simulink model "AM_FM"  (R2023a)
settings: Solver=VariableStepAuto  StartTime=0.0  StopTime=0.5  RelTol=1e-3
libraries: commanabbnd3 x4, dspfdesign x1, commsynccomp2 x1
settings Model: SimulationMode=accelerator  Creator=moleiva  LastModifiedBy=luisc
settings ModelReferenceCC: EnableRefExpFcnMdlSchedulingChecks=on

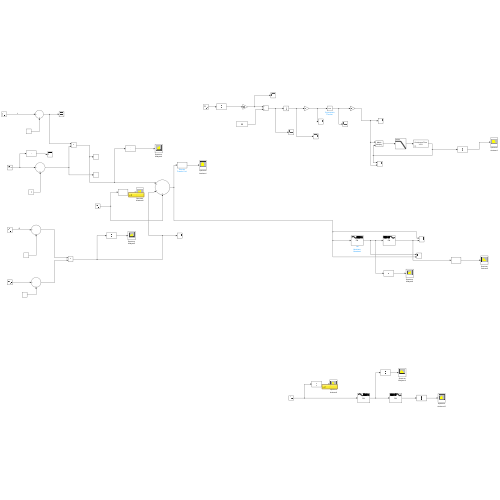
[thumbnail: Simulink's stored preview of the top-level diagram]
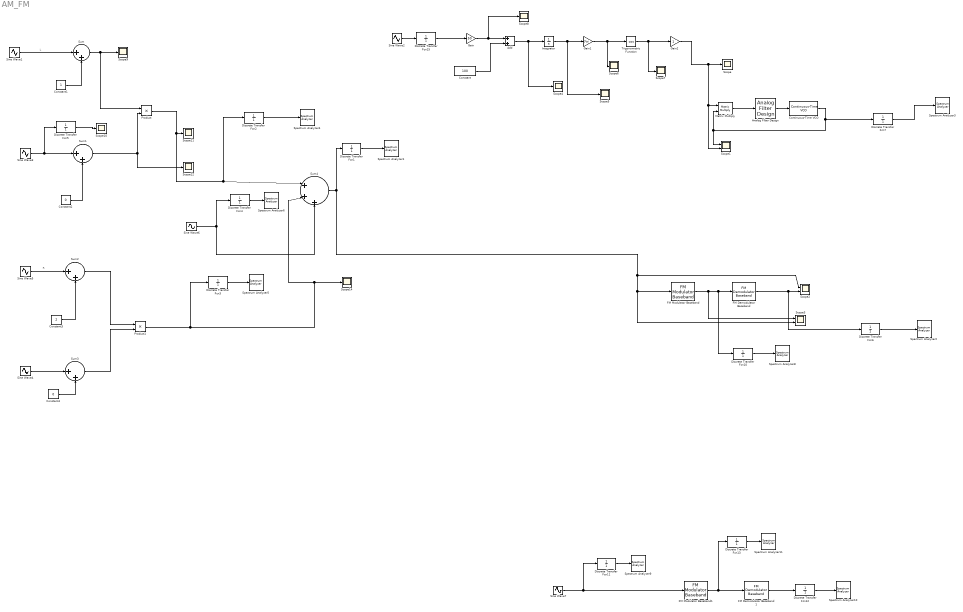
== system AM_FM ==
  note: R
  note: L
  Add : Sum
  Analog Filter Design : dspfdesign/Analog Filter Design  method=Butterworth  filttype=Lowpass  N=8  Wlo=20e+6  Whi=80  Rp=2  Rs=40
  Constant : Constant  Value=100  VectorParams1D=off
  Constant1 : Constant
  Constant2 : Constant  Value=0
  Constant3 : Constant  Value=2
  Constant4 : Constant  Value=0
  Continuous-Time VCO : commsynccomp2/Continuous-Time VCO  Ac=1  Fc=10  Kc=1  Ph=0
  Discrete Transfer Fcn1 : DiscreteTransferFcn  Denominator=[1]  SampleTime=1/24e+6
  Discrete Transfer Fcn{2,5..6,10,12} (5 alike) : DiscreteTransferFcn  Denominator=[1]  SampleTime=1/16e+6
  Discrete Transfer Fcn11 : DiscreteTransferFcn  Denominator=[1]  SampleTime=1/12e+6
  Discrete Transfer Fcn13 : DiscreteTransferFcn  Denominator=[1]  SampleTime=1/12e+6
  Discrete Transfer Fcn15 : DiscreteTransferFcn  Denominator=[1]  SampleTime=1/2*pi*100
  Discrete Transfer Fcn3 : DiscreteTransferFcn  Denominator=[1]  SampleTime=1/24e+6
  Discrete Transfer Fcn4 : DiscreteTransferFcn  Denominator=[1]  SampleTime=1/12e+6
  Discrete Transfer Fcn7 : DiscreteTransferFcn  Denominator=[1]  SampleTime=1/200
  "FM Demodulator Baseband " : commanabbnd3/FM Demodulator Baseband   FrequencyDeviation=50  SimulateUsing=Code generation
  FM Demodulator Baseband 1 : commanabbnd3/FM Demodulator Baseband   FrequencyDeviation=50  SimulateUsing=Code generation
  FM Modulator Baseband : commanabbnd3/FM Modulator Baseband  FrequencyDeviation=50  SimulateUsing=Code generation
  FM Modulator Baseband1 : commanabbnd3/FM Modulator Baseband  FrequencyDeviation=50  SimulateUsing=Code generation
  Gain : Gain  Gain=50
  Gain1 : Gain  Gain=2*pi
  Gain2 : Gain
  Integrator : Integrator
  Matrix Multiply : Product  Multiplication=Matrix(*)
  Product : Product
  Product1 : Product
  Scope{,4..12,14} (11 alike) : Scope
  Scope1 : Scope  NumInputPorts=2
  Scope2 : Scope  NumInputPorts=2
  Scope3 : Scope  NumInputPorts=2
  Sine Wave1 : Sin  Frequency=2*pi*5000  Phase=pi/2  SampleTime=0  VectorParams1D=off
  Sine Wave2 : Sin  Frequency=2*pi*50  Phase=pi/2  SampleTime=0  VectorParams1D=off
  Sine Wave3 : Sin  Frequency=2*pi*8e+6  Phase=pi/2  SampleTime=0  VectorParams1D=off
  Sine Wave4 : Sin  Frequency=2*pi*12e+6  Phase=pi/2  SampleTime=0  VectorParams1D=off
  Sine Wave5 : Sin  Frequency=2*pi*4000  Phase=pi/2  SampleTime=0  VectorParams1D=off
  Sine Wave6 : Sin  Amplitude=2  Frequency=2*pi*6e+6  Phase=pi/2  SampleTime=0  VectorParams1D=off
  Sine Wave7 : Sin  Amplitude=2  Frequency=2*pi*6e+6  Phase=pi/2  SampleTime=0  VectorParams1D=off
  Spectrum Analyzer1 : SpectrumAnalyzer  WindowPosition=[1.000000,41.000000,1536.000000,801.000000,]  ScopeFrameLocation=window  AxesScaling=Manual  AveragingMethod=Exponential  SpectrumUnits=Watts  YLimits=[-0.51276374,4.61487369]  ShowLegend=on  ChannelNames="[\"\"]"  SelectedToolstripTab=spectrumAnalyzerToolstrip.spectrumTab  DefaultConfigurationName=spbscopes.SpectrumAnalyzerBlockCfg
      settings: OpenAtSimulationStart=off
  Spectrum Analyzer10 : SpectrumAnalyzer  WindowPosition=[770.000000,42.000000,766.000000,793.000000,]  Visible=on  ScopeFrameLocation=window  AxesScaling=Manual  AveragingMethod=Exponential  YLimits=[-73.15760482,41.44536822]  ChannelNames="[\"\"]"  DefaultConfigurationName=spbscopes.SpectrumAnalyzerBlockCfg
      settings: OpenAtSimulationStart=off
  Spectrum Analyzer11 : SpectrumAnalyzer  WindowPosition=[2.000000,42.000000,766.000000,793.000000,]  Visible=on  ScopeFrameLocation=window  AxesScaling=Manual  AveragingMethod=Exponential  YLimits=[-74.13776805,40.75747711]  ChannelNames="[\"\"]"  DefaultConfigurationName=spbscopes.SpectrumAnalyzerBlockCfg
      settings: OpenAtSimulationStart=off
  Spectrum Analyzer2 : SpectrumAnalyzer  WindowPosition=[1.000000,41.000000,1536.000000,801.000000,]  Visible=on  ScopeFrameLocation=window  AxesScaling=Manual  AveragingMethod=Exponential  YLimits=[-221.40437999,59.98570956]  ChannelNames="[\"\"]"  DefaultConfigurationName=spbscopes.SpectrumAnalyzerBlockCfg
      settings: OpenAtSimulationStart=off
  Spectrum Analyzer3 : SpectrumAnalyzer  WindowPosition=[1.000000,41.000000,1536.000000,801.000000,]  ScopeFrameLocation=window  AxesScaling=Manual  AveragingMethod=Exponential  SpectrumUnits=Watts  YLimits=[-123.17973841,46.92856517]  ChannelNames="[\"\"]"  SelectedToolstripTab=spectrumAnalyzerToolstrip.spectrumTab  DefaultConfigurationName=spbscopes.SpectrumAnalyzerBlockCfg
      settings: OpenAtSimulationStart=off
  Spectrum Analyzer4 : SpectrumAnalyzer  WindowPosition=[1.000000,1.000000,1536.000000,841.000000,]  ScopeFrameLocation=window  AxesScaling=Manual  AveragingMethod=Exponential  YLimits=[-149.30305087,57.1601735]  ChannelNames="[\"\"]"  DefaultConfigurationName=spbscopes.SpectrumAnalyzerBlockCfg
      settings: OpenAtSimulationStart=off
  Spectrum Analyzer5 : SpectrumAnalyzer  WindowPosition=[368.000000,182.000000,800.000000,500.000000,]  ScopeFrameLocation=window  AxesScaling=Manual  AveragingMethod=Exponential  ChannelNames="[\"\"]"  DefaultConfigurationName=spbscopes.SpectrumAnalyzerBlockCfg
      settings: OpenAtSimulationStart=off
  Spectrum Analyzer6 : SpectrumAnalyzer  WindowPosition=[368.000000,182.000000,800.000000,500.000000,]  ScopeFrameLocation=window  AxesScaling=Manual  AveragingMethod=Exponential  ChannelNames="[\"\"]"  DefaultConfigurationName=spbscopes.SpectrumAnalyzerBlockCfg
      settings: OpenAtSimulationStart=off
  Spectrum Analyzer8 : SpectrumAnalyzer  WindowPosition=[2.000000,42.000000,1534.000000,793.000000,]  ScopeFrameLocation=window  AxesScaling=Manual  AveragingMethod=Exponential  YLimits=[-117.39798875,29.52252221]  ChannelNames="[\"\"]"  DefaultConfigurationName=spbscopes.SpectrumAnalyzerBlockCfg
      settings: OpenAtSimulationStart=off
  Spectrum Analyzer9 : SpectrumAnalyzer  WindowPosition=[90.000000,154.000000,800.000000,500.000000,]  ScopeFrameLocation=window  AxesScaling=Manual  AveragingMethod=Exponential  ChannelNames="[\"\"]"  DefaultConfigurationName=spbscopes.SpectrumAnalyzerBlockCfg
      settings: OpenAtSimulationStart=off
  Sum{,1..3} (4 alike) : Sum  Inputs=|++
  Sum4 : Sum  Inputs=|+++
  Trigonometric Function : Trigonometry  Operator=cos
  wires:
  Gain/1 -> Scope8/1, Add/1
  Add/1 -> Scope4/1, Integrator/1
  Integrator/1 -> Scope5/1, Gain1/1
  Gain1/1 -> Scope6/1, Trigonometric Function/1
  Trigonometric Function/1 -> Scope7/1, Gain2/1
  Constant/1 -> Add/2
  Gain2/1 -> Scope1/2, Matrix Multiply/1, Scope/1
  Matrix Multiply/1 -> Analog Filter Design/1
  Analog Filter Design/1 -> Continuous-Time VCO/1
  Sum4/1 -> Scope3/2, FM Modulator Baseband/1, Scope2/1, Discrete Transfer Fcn1/1
  FM Modulator Baseband/1 -> Scope3/1, Discrete Transfer Fcn10/1, "FM Demodulator Baseband "/1
  "FM Demodulator Baseband "/1 -> Discrete Transfer Fcn6/1, Scope2/2
  Sum3/1 -> Product1/2
  Discrete Transfer Fcn2/1 -> Spectrum Analyzer4/1
  Discrete Transfer Fcn5/1 -> Scope10/1
  Discrete Transfer Fcn1/1 -> Spectrum Analyzer1/1
  Sum1/1 -> Product/2, Scope12/1
  Sum/1 -> Product/1, Scope9/1
  Discrete Transfer Fcn3/1 -> Spectrum Analyzer5/1
  Constant3/1 -> Sum2/2
  Constant1/1 -> Sum/2
  Sine Wave4/1 -> Sum3/1
  Constant4/1 -> Sum3/2
  Sine Wave5/1 -> Sum2/1
  Sine Wave3/1 -> Discrete Transfer Fcn5/1, Sum1/1
  Constant2/1 -> Sum1/2
  Sine Wave1/1 -> Sum/1
  Product1/1 -> Discrete Transfer Fcn3/1, Sum4/2, Scope14/1
  Discrete Transfer Fcn4/1 -> Spectrum Analyzer6/1
  Sum2/1 -> Product1/1
  Product/1 -> Discrete Transfer Fcn2/1, Sum4/1, Scope11/1
  Discrete Transfer Fcn6/1 -> Spectrum Analyzer2/1
  Continuous-Time VCO/1 -> Scope1/1, Matrix Multiply/2, Discrete Transfer Fcn7/1
  Discrete Transfer Fcn7/1 -> Spectrum Analyzer3/1
  Sine Wave6/1 -> Sum4/3, Discrete Transfer Fcn4/1
  Discrete Transfer Fcn10/1 -> Spectrum Analyzer8/1
  Sine Wave7/1 -> FM Modulator Baseband1/1, Discrete Transfer Fcn11/1
  Discrete Transfer Fcn11/1 -> Spectrum Analyzer9/1
  FM Modulator Baseband1/1 -> Discrete Transfer Fcn13/1, FM Demodulator Baseband 1/1
  Discrete Transfer Fcn12/1 -> Spectrum Analyzer10/1
  FM Demodulator Baseband 1/1 -> Discrete Transfer Fcn12/1
  Discrete Transfer Fcn13/1 -> Spectrum Analyzer11/1
  Discrete Transfer Fcn15/1 -> Gain/1
  Sine Wave2/1 -> Discrete Transfer Fcn15/1
